simulink model "Autopilot_q_running1"  (R2021a)
settings: Solver=ode4  StartTime=0.0  StopTime=168  FixedStep=0.01  RelTol=1e-3
undefined symbols (not defined in the file or in its folder): Aero_cofficients, Earth, Plane_state_store, Structural_data, Thrust_data_store, WGS84
libraries: pid_lib x12, aerolibactuator x5, aerolibfltsims x2, aerolibanim x1, simulink x1, aerolibtransform2 x1, shared6dof x1, sim3dlib x1, uavsim3dlib x1
(part 1 of 3)
settings Model: PauseTimes=.01  Creator=rrpat  LastModifiedBy=PC
settings SolverCC: AlgebraicLoopSolver=LineSearch
settings DataIOCC: ReturnWorkspaceOutputs=off
settings DebuggingCC: SFMachineParentedDataDiag=warning  ArithmeticOperatorsInVariantConditions=warning
settings SFSimCC: CustomCodeUndefinedFunction=UseInterfaceOnly

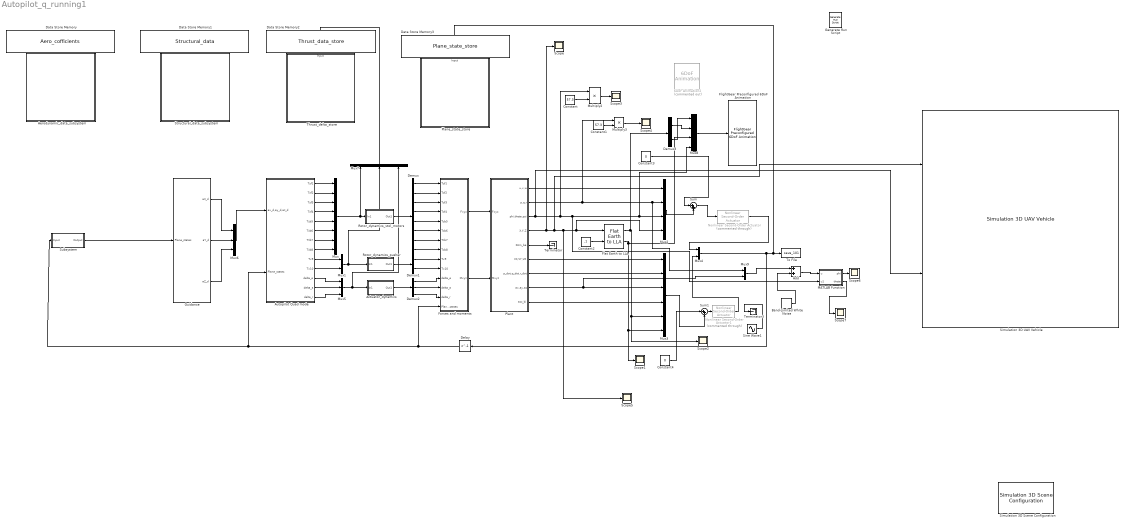
== system Autopilot_q_running1 ==
  6DoF Animation2 : aerolibanim/6DoF Animation  Commented=on  u1=[-150 150 -150 150 -150 150]  u2=0.1  u3=100  u4=[-4000 0 2000]  u5=Fly alongside  u6="[300  300 -200]"  u7=10  u8=on
  Actuator_dynamics : Subsystem
  Add : Sum
  Aerodynamic_data_subsystem : Subsystem
  Autopilot Quad mode : Subsystem
  Band-Limited White Noise : simulink/Sources/Band-Limited White Noise  Cov=[0.0001]  Ts=0.1  seed=[23341]
  Constant : Constant  Value=57.3
  Constant1 : Constant  Value=57.3
  Constant2 : Constant  Value=-7
  Constant3 : Constant  Value=0
  Constant4 : Constant  Value=0
  Data Store Memory : DataStoreMemory  DataStoreName=Aero_cofficients  ReadBeforeWriteMsg=warning  WriteAfterWriteMsg=warning  WriteAfterReadMsg=warning  InitialValue=[0 0 0 0 0 0 0 0 0;0 0 0 0 0 0 0 0 0;0 0 0 0 0 0 0 0 0;0 0 0 0 0 0 0 0 0;0 0 0 0 0 0 0 0 0;0 0 0 0 0 0 0 0 0]  ShareAcrossModelInstances=on  VectorParams1D=off  ShowAdditionalParam=off
  Data Store Memory1 : DataStoreMemory  DataStoreName=Structural_data  ReadBeforeWriteMsg=warning  WriteAfterWriteMsg=warning  WriteAfterReadMsg=warning  InitialValue=[25.0,0,0,0,0,0,0,0,0,0,0,0,0,0,0,0,0,0,0,0,0,0,0,0]  ShareAcrossModelInstances=on  VectorParams1D=off  ShowAdditionalParam=off
  Data Store Memory2 : DataStoreMemory  DataStoreName=Thrust_data_store  ReadBeforeWriteMsg=warning  WriteAfterWriteMsg=warning  WriteAfterReadMsg=warning  InitialValue=[0,0,0,0,0,0,0,0,0,0,0,0,0]  ShareAcrossModelInstances=on  VectorParams1D=off  ShowAdditionalParam=off
  Data Store Memory3 : DataStoreMemory  DataStoreName=Plane_state_store  ReadBeforeWriteMsg=warning  WriteAfterWriteMsg=warning  WriteAfterReadMsg=warning  InitialValue=[0.0,0,0,0,0,0,0,0,30/57.3,0,0,0,0,0,0,0,0,0,0,0,0,0,0,0,0,0,0]  ShareAcrossModelInstances=on  VectorParams1D=off  ShowAdditionalParam=off
  Delay : Delay  DelayLength=1
  Demux : Demux  Outputs=8
  Demux1 : Demux  Outputs=2
  Demux2 : Demux  Outputs=3
  Demux3 : Demux  Outputs=2
  Flat Earth to LLA : aerolibtransform2/Flat Earth to LLA  units=Metric (MKS)  ptype=Earth (WGS84)  F=1/298.257223563  R=6378137  refPosPort=off  LL0=[37.6188056,-122.3754167 ]  psi=0
  FlightGear Preconfigured 6DoF Animation : aerolibfltsims/FlightGear Preconfigured 6DoF Animation  xFlightGearVersion=v2016.3  DestinationIpAddress=127.0.0.1  DestinationPort=5502  SampleTime=0.01  packetVersion=24
  Forces and moments : Subsystem
  Generate Run Script : aerolibfltsims/Generate Run Script  Architecture=Default  dataFlow=Send  GeometryModelName=HL20  AirportId=KSFO  RunwayId=10L  InitialAltitude=500  InitialHeading=0  OffsetDistance=4.72  OffsetAzimuth=0  InstallScenery=on  DisableShaders=off  OriginAddress=127.0.0.1  DestinationPort=5502  OriginPort=5505  LocalAddress=127.0.0.1  OutputFileName=runfg.bat  FlightGearBaseDirectory=C:\Program Files\FlightGear 2016.3.1
  Guidance : Subsystem
  MATLAB Function : MATLAB Function  TreatAsAtomicUnit=on
  Multiply2 : Product
  Multiply3 : Product
  Mux : Mux  Inputs=8
  Mux1 : Mux  Inputs=2
  Mux2 : Mux
  Mux3 : Mux  Inputs=6
  Mux4 : Mux  Inputs=2
  Mux5 : Mux  Inputs=3
  Mux6 : Mux  Inputs=3
  Mux7 : Mux  Inputs=3
  Mux8 : Mux
  Mux9 : Mux  Inputs=2
  Nonlinear Second-Order Actuator : aerolibactuator/Nonlinear Second-Order Actuator  Commented=through  wn_fin=50  z_fin=0.5  fin_max=500000000  fin_min=-500000000  fin_maxrate=2  fin_act_0=0  fin_act_vel=0
      settings: SourceProductBaseCode=AE
  Nonlinear Second-Order Actuator1 : aerolibactuator/Nonlinear Second-Order Actuator  Commented=through  wn_fin=50  z_fin=0.5  fin_max=5000000  fin_min=-5000000  fin_maxrate=2  fin_act_0=0  fin_act_vel=0
      settings: SourceProductBaseCode=AE
  Plane_state_store : Subsystem
  Plant : Subsystem
  Rotor_dynamics_pusher : Subsystem
  Rotor_dynamics_vtol_motors : Subsystem
  Scope{,1..7} (8 alike) : Scope
  Simulation 3D Scene Configuration : sim3dlib/Simulation 3D Scene Configuration  Priority=0  ProjectFormat=Default Scenes  SceneDesc=US city block  ProjectName=C:\Program Files\MATLAB\R2021a\toolbox\shared\sim3d_projects\automotive_project\UE4\WindowsNoEditor\VehicleSimulation.exe  ScenePath=/Game/Maps/HwStrght  vehTagList={'Scene Origin';'SimulinkVehicle1'}  vehTag=SimulinkVehicle1  OpVisEn=off  Ts=0.01  EnableWindow=on  EnableWeather=off  SunAltitude=40.0  SunAzimuth=90  clouds=10  wind=1  fog=0  rain=0  sensorTag=MainCamera1  sensorId=1  sensorName=MainCamera1  mountLoc=Origin  offsetFlag=off  tmountOffset=[0, 0, 0]  rmountOffset=[0, 0, 0]  HorizontalResolution=1280  VerticalResolution=720  HorizontalFOV=60  mountPoint=[0 0 0]  mountOrientation=[0 0 0]  aMode=3  ID=1
      settings: SourceProductBaseCode=DR,UV,VE
  Simulation 3D UAV Vehicle : uavsim3dlib/Simulation 3D UAV Vehicle  Priority=-1  Mesh=Quadrotor  Color=Blue  ActorName=SimulinkVehicle1  InitialTranslation=[0 0 0]  InitialRotation=[0 0 0]  SampleTime=-1  ActorType=SimulinkVehicle  ID=1  aMode=4  ActorTag=SimulinkVehicle1
      settings: SourceProductBaseCode=UV
  Sine Wave1 : Sin  Amplitude=0.1/57.3  Frequency=100*2*3.1415  SampleTime=0
  Structural_data_subsystem : Subsystem
  Subsystem : Subsystem
  Sum : Sum  Inputs=|++
  Sum1 : Sum  Inputs=|++
  Terminator : Terminator
  Terminator3 : Terminator
  Thrust_delta_store : Subsystem
  To File : ToFile  Filename=save_101  SaveFormat=Timeseries
  wires:
  Constant2/1 -> Flat Earth to LLA/2
  Plant/4(X,Y,Z) -> Scope/1, Simulation 3D UAV Vehicle/1, Scope5/1, Mux2/4, Flat Earth to LLA/1
  Plant/5(Dcm_be) -> Terminator/1
  Plant/1(u,v,w) -> Mux2/1
  Plant/2(p,q,r) -> Multiply3/1, Mux9/1, Mux2/2
  Plant/3(phi,theta,psi) -> Simulation 3D UAV Vehicle/2, MATLAB Function/2(u1), Mux8/4, Mux2/3, Multiply2/1
  Plant/9(acc_bi) -> Mux3/4
  Plant/8(ax,ay,az) -> Mux9/2, Mux3/3
  Plant/7(p_dot,q_dot,r_dot) -> Mux3/2
  Plant/6(VX,VY,VZ) -> Mux3/1
  Forces and moments/2(Mxyz) -> Plant/2(Mxyz)
  Flat Earth to LLA/1 -> Demux3/1, Mux3/5, Scope2/1
  Flat Earth to LLA/2 -> Mux8/3, Mux3/6, Scope1/1
  Autopilot Quad mode/1(Tzf1) -> Mux/1
  Autopilot Quad mode/2(Tzf2) -> Mux/2
  Autopilot Quad mode/3(Tzf3) -> Mux/3
  Autopilot Quad mode/4(Tzf4) -> Mux/4
  Autopilot Quad mode/5(Tzb5) -> Mux/5
  Autopilot Quad mode/6(Tzb6) -> Mux/6
  Autopilot Quad mode/7(Tzb7) -> Mux/7
  Autopilot Quad mode/8(Tzb8) -> Mux/8
  Demux/8 -> Forces and moments/8(Tzb8)
  Demux/7 -> Forces and moments/7(Tzb7)
  Demux/1 -> Forces and moments/1(Tzf1)
  Demux/3 -> Forces and moments/3("Tzf3 ")
  Demux/4 -> Forces and moments/4(Tzf4)
  Demux/5 -> Forces and moments/5(Tzb5)
  Demux/6 -> Forces and moments/6(Tzb6)
  Demux1/1 -> Forces and moments/9(Tx9)
  Demux1/2 -> Forces and moments/10(Tx10)
  Rotor_dynamics_pusher/1(Out1) -> Demux1/1
  Autopilot Quad mode/9(Tx9) -> Mux1/1
  Autopilot Quad mode/10(Tx10) -> Mux1/2
  Demux2/1 -> Forces and moments/11(delta_e)
  Demux2/2 -> Forces and moments/12(delta_a)
  Demux2/3 -> Forces and moments/13(delta_r)
  Actuator_dynamics/1(Out1) -> Demux2/1
  Autopilot Quad mode/11(delta_e) -> Mux5/1
  Autopilot Quad mode/12(delta_a) -> Mux5/2
  Autopilot Quad mode/13(delta_r) -> Mux5/3
  Rotor_dynamics_vtol_motors/1(Out1) -> Demux/1
  Forces and moments/1(Fxyz) -> Plant/1(Fxyz)
  Guidance/1(aX_d) -> Mux6/1
  Guidance/3(aZ_d) -> Mux6/3
  Guidance/2(aY_d) -> Mux6/2
  Mux6/1 -> Autopilot Quad mode/1(ax_d,ay_d,az_d)
  Mux/1 -> Mux7/1, Rotor_dynamics_vtol_motors/1(In1)
  Mux1/1 -> Rotor_dynamics_pusher/1(In1), Mux7/2
  Mux5/1 -> Actuator_dynamics/1(In1), Mux7/3
  Subsystem/1(Output) -> Guidance/1(Plane_states)
  Mux7/1 -> Thrust_delta_store/1(Input)
  Constant/1 -> Multiply2/2
  Multiply2/1 -> Scope3/1
  Constant1/1 -> Multiply3/2
  Multiply3/1 -> Scope4/1
  Mux3/1 -> Sum1/2
  Mux2/1 -> Sum/2
  Sine Wave1/1 -> Terminator3/1
  Sum/1 -> Nonlinear Second-Order Actuator/1
  Mux4/1 -> Plane_state_store/1(Input), To File/1, Delay/1
  Sum1/1 -> Nonlinear Second-Order Actuator1/1
  Nonlinear Second-Order Actuator/1 -> Mux4/1
  Nonlinear Second-Order Actuator1/1 -> Mux4/2
  Mux8/1 -> FlightGear Preconfigured 6DoF Animation/1
  Demux3/1 -> Mux8/2
  Constant3/1 -> Sum/1
  Constant4/1 -> Sum1/1
  Demux/2 -> Forces and moments/2(Tzf2)
  Demux3/2 -> Mux8/1
  Mux9/1 -> Add/1
  Band-Limited White Noise/1 -> Add/2
  Add/1 -> MATLAB Function/1(u)
  MATLAB Function/1(phi) -> Scope6/1
  MATLAB Function/2(theta) -> Scope7/1
  Delay/1 -> Subsystem/1(Input), Autopilot Quad mode/2(Plane_states), Forces and moments/14(Plane_states)

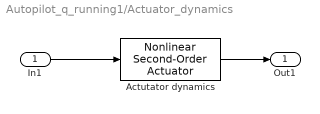
== system Autopilot_q_running1/Actuator_dynamics ==
  In1 : Inport
  Actutator dynamics : aerolibactuator/Nonlinear Second-Order Actuator  wn_fin=100  z_fin=0.3  fin_max=20*pi/180  fin_min=-20*pi/180  fin_maxrate=500*pi/180  fin_act_0=0  fin_act_vel=0
      settings: SourceProductBaseCode=AE
  Out1 : Outport  VectorParamsAs1DForOutWhenUnconnected=off
  wires:
  Actutator dynamics/1 -> Out1/1
  In1/1 -> Actutator dynamics/1

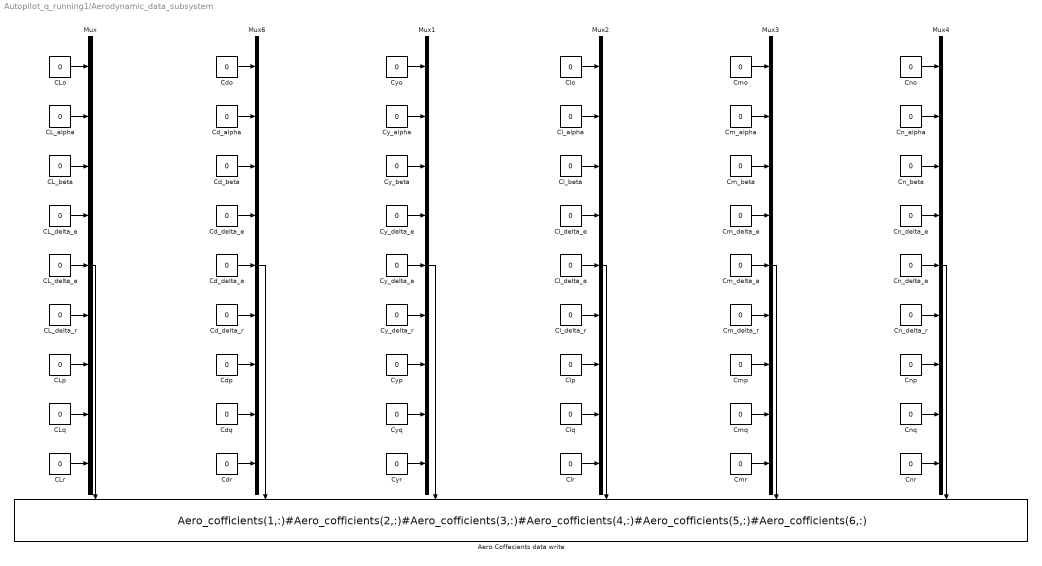
== system Autopilot_q_running1/Aerodynamic_data_subsystem ==
  Aero Coffecients data write : DataStoreWrite  DataStoreName=Aero_cofficients  DataStoreElements=Aero_cofficients(1,:)#Aero_cofficients(2,:)#Aero_cofficients(3,:)#Aero_cofficients(4,:)#Aero_cofficients(5,:)#Aero_cofficients(6,:)  IndexOptions=Index vector (dialog)  Indices=1  OutputSizes=1
  CL_alpha : Constant  Value=0
  CL_beta : Constant  Value=0
  CL_delta_a : Constant  Value=0
  CL_delta_e : Constant  Value=0
  CL_delta_r : Constant  Value=0
  CLo : Constant  Value=0
  CLp : Constant  Value=0
  CLq : Constant  Value=0
  CLr : Constant  Value=0
  Cd_alpha : Constant  Value=0
  Cd_beta : Constant  Value=0
  Cd_delta_a : Constant  Value=0
  Cd_delta_e : Constant  Value=0
  Cd_delta_r : Constant  Value=0
  Cdo : Constant  Value=0
  Cdp : Constant  Value=0
  Cdq : Constant  Value=0
  Cdr : Constant  Value=0
  Cl_alpha : Constant  Value=0
  Cl_beta : Constant  Value=0
  Cl_delta_a : Constant  Value=0
  Cl_delta_e : Constant  Value=0
  Cl_delta_r : Constant  Value=0
  Clo : Constant  Value=0
  Clp : Constant  Value=0
  Clq : Constant  Value=0
  Clr : Constant  Value=0
  Cm_alpha : Constant  Value=0
  Cm_beta : Constant  Value=0
  Cm_delta_a : Constant  Value=0
  Cm_delta_e : Constant  Value=0
  Cm_delta_r : Constant  Value=0
  Cmo : Constant  Value=0
  Cmp : Constant  Value=0
  Cmq : Constant  Value=0
  Cmr : Constant  Value=0
  Cn_alpha : Constant  Value=0
  Cn_beta : Constant  Value=0
  Cn_delta_a : Constant  Value=0
  Cn_delta_e : Constant  Value=0
  Cn_delta_r : Constant  Value=0
  Cno : Constant  Value=0
  Cnp : Constant  Value=0
  Cnq : Constant  Value=0
  Cnr : Constant  Value=0
  Cy_alpha : Constant  Value=0
  Cy_beta : Constant  Value=0
  Cy_delta_a : Constant  Value=0
  Cy_delta_e : Constant  Value=0
  Cy_delta_r : Constant  Value=0
  Cyo : Constant  Value=0
  Cyp : Constant  Value=0
  Cyq : Constant  Value=0
  Cyr : Constant  Value=0
  Mux{,1..4,6} (6 alike) : Mux  Inputs=9
  wires:
  Mux/1 -> Aero Coffecients data write/1
  CLo/1 -> Mux/1
  CL_alpha/1 -> Mux/2
  CL_beta/1 -> Mux/3
  CL_delta_e/1 -> Mux/4
  CL_delta_a/1 -> Mux/5
  CL_delta_r/1 -> Mux/6
  CLp/1 -> Mux/7
  CLq/1 -> Mux/8
  CLr/1 -> Mux/9
  Cdo/1 -> Mux6/1
  Cd_delta_e/1 -> Mux6/4
  Cdq/1 -> Mux6/8
  Cdp/1 -> Mux6/7
  Cd_delta_a/1 -> Mux6/5
  Cdr/1 -> Mux6/9
  Cd_beta/1 -> Mux6/3
  Cd_delta_r/1 -> Mux6/6
  Cd_alpha/1 -> Mux6/2
  Mux6/1 -> Aero Coffecients data write/2
  Cy_alpha/1 -> Mux1/2
  Cy_delta_r/1 -> Mux1/6
  Cy_beta/1 -> Mux1/3
  Cyr/1 -> Mux1/9
  Cy_delta_a/1 -> Mux1/5
  Cyp/1 -> Mux1/7
  Cyq/1 -> Mux1/8
  Cy_delta_e/1 -> Mux1/4
  Cyo/1 -> Mux1/1
  Mux1/1 -> Aero Coffecients data write/3
  Mux2/1 -> Aero Coffecients data write/4
  Clo/1 -> Mux2/1
  Cl_delta_e/1 -> Mux2/4
  Clq/1 -> Mux2/8
  Clp/1 -> Mux2/7
  Cl_delta_a/1 -> Mux2/5
  Clr/1 -> Mux2/9
  Cl_beta/1 -> Mux2/3
  Cl_delta_r/1 -> Mux2/6
  Cl_alpha/1 -> Mux2/2
  Mux3/1 -> Aero Coffecients data write/5
  Cmo/1 -> Mux3/1
  Cm_delta_e/1 -> Mux3/4
  Cmq/1 -> Mux3/8
  Cmp/1 -> Mux3/7
  Cm_delta_a/1 -> Mux3/5
  Cmr/1 -> Mux3/9
  Cm_beta/1 -> Mux3/3
  Cm_delta_r/1 -> Mux3/6
  Cm_alpha/1 -> Mux3/2
  Mux4/1 -> Aero Coffecients data write/6
  Cno/1 -> Mux4/1
  Cn_delta_e/1 -> Mux4/4
  Cnq/1 -> Mux4/8
  Cnp/1 -> Mux4/7
  Cn_delta_a/1 -> Mux4/5
  Cnr/1 -> Mux4/9
  Cn_beta/1 -> Mux4/3
  Cn_delta_r/1 -> Mux4/6
  Cn_alpha/1 -> Mux4/2

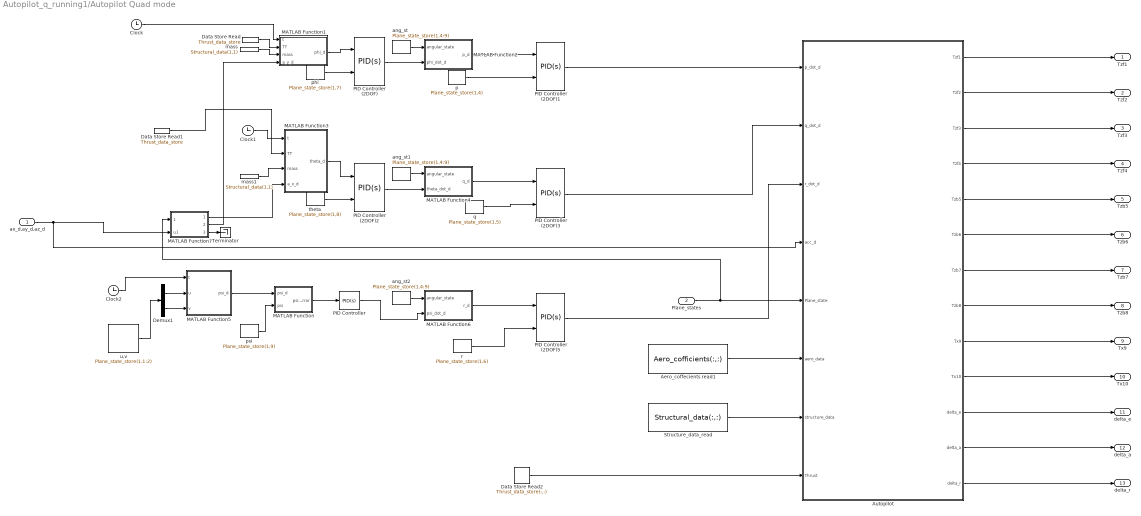
== system Autopilot_q_running1/Autopilot Quad mode ==
  ax_d,ay_d,az_d : Inport
  Plane_states : Inport  Port=2
  Aero_coffecients read1 : DataStoreRead  DataStoreName=Aero_cofficients  DataStoreElements=Aero_cofficients(:,:)  IndexOptions=Index vector (dialog)  Indices=1  OutputSizes=1
  Autopilot : MATLAB Function  TreatAsAtomicUnit=on
  Clock : Clock
      settings: Decimation=200
  Clock1 : Clock
      settings: Decimation=200
  Clock2 : Clock
      settings: Decimation=200
  Data Store Read : DataStoreRead  DataStoreName=Thrust_data_store  IndexOptions=Index vector (dialog)  Indices=1  OutputSizes=1
  Data Store Read1 : DataStoreRead  DataStoreName=Thrust_data_store  IndexOptions=Index vector (dialog)  Indices=1  OutputSizes=1
  Data Store Read2 : DataStoreRead  DataStoreName=Thrust_data_store  DataStoreElements=Thrust_data_store(:,:)  IndexOptions=Index vector (dialog)  Indices=1  OutputSizes=1
  Demux1 : Demux  Outputs=2
  MATLAB Function : MATLAB Function  TreatAsAtomicUnit=on
  MATLAB Function1 : MATLAB Function  TreatAsAtomicUnit=on
  MATLAB Function2 : MATLAB Function  TreatAsAtomicUnit=on
  MATLAB Function3 : MATLAB Function  TreatAsAtomicUnit=on
  MATLAB Function4 : MATLAB Function  TreatAsAtomicUnit=on
  MATLAB Function5 : MATLAB Function  TreatAsAtomicUnit=on
  MATLAB Function6 : MATLAB Function  TreatAsAtomicUnit=on
  MATLAB Function7 : MATLAB Function  TreatAsAtomicUnit=on
  PID Controller : pid_lib/PID Controller  Controller=PID  Form=Parallel  TimeDomain=Continuous-time  UseExternalTs=off  SampleTime=-1  IntegratorMethod=Forward Euler  FilterMethod=Forward Euler  ControllerParametersSource=internal  P=1  I=0  D=0  UseFilter=on  N=100  TunerSelectOption=Transfer Function Based (PID Tuner App)  InitialConditionSource=internal  InitialConditionForIntegrator=0  InitialConditionForFilter=0  DifferentiatorICPrevScaledInput=0  ExternalReset=none  TrackingMode=off  Kt=1  LimitOutput=off  SatLimitsSource=internal  UpperSaturationLimit=inf  LowerSaturationLimit=-inf  LinearizeAsGain=on  AntiWindupMode=none  Kb=1  POutMin=[]  POutMax=[]  IOutMin=[]  IOutMax=[]  DOutMin=[]  DOutMax=[]  NOutMin=[]  NOutMax=[]  SumOutMin=[]  SumOutMax=[]  SaturationOutMin=[]  SaturationOutMax=[]  PParamMin=[]  PParamMax=[]  IParamMin=[]  IParamMax=[]  DParamMin=[]  DParamMax=[]  NParamMin=[]  NParamMax=[]  KbParamMin=[]  KbParamMax=[]  KtParamMin=[]  KtParamMax=[]  KbOutMin=[]  KbOutMax=[]  KtOutMin=[]  KtOutMax=[]  IntegratorOutMin=[]  IntegratorOutMax=[]  FilterOutMin=[]  FilterOutMax=[]  SumI1OutMin=[]  SumI1OutMax=[]  SumI2OutMin=[]  SumI2OutMax=[]  SumI3OutMin=[]  SumI3OutMax=[]  SumI4OutMin=[]  SumI4OutMax=[]  SumDOutMin=[]  SumDOutMax=[]  DifferentiatorOutMin=[]  DifferentiatorOutMax=[]  FilterDiffOutCoefMin=[]  FilterDiffOutCoefMax=[]  ReciprocalOutMin=[]  ReciprocalOutMax=[]  SumDenOutMin=[]  SumDenOutMax=[]  SumNumOutMin=[]  SumNumOutMax=[]  DivideOutMin=[]  DivideOutMax=[]  UdiffTsProdOutMin=[]  UdiffTsProdOutMax=[]  NTsProdOutMin=[]  NTsProdOutMax=[]  UintegralTsProdOutMin=[]  UintegralTsProdOutMax=[]  UngainTsProdOutMin=[]  UngainTsProdOutMax=[]  IntegratorContinuousStateAttributes=''  IntegratorStateMustResolveToSignalObject=off  IntegratorRTWStateStorageClass=Auto  FilterContinuousStateAttributes=''  FilterStateMustResolveToSignalObject=off  FilterRTWStateStorageClass=Auto  ParallelPVariant=InternalParameters  IdealPVariant=Disabled  IVariant=InternalParameters  DVariant=InternalParameters  IntegratorVariant=Continuous  SatVariant=Disabled  AWVariant=Passthrough  PCopyVariant=Disabled  TRVariant=Disabled  FdbkBlocksVariant=Forward  IdealPFdbkVariant=Disabled  SatFdbkVariant=Disabled  DerivativeFilterVariant=ContFilter  NVariant=InternalParameters  NCopyVariant=Disabled  FilterICVariant=InternalICsFilter  IntegratorICVariant=InternalICs  ExternalResetVariant=Disabled  TRSumVariant=Passthrough  SumFdbkVariant=Disabled  SumVariant=Sum_PID  TsampFilterVariant=InternalTs  TsampNgainVariant=Passthrough  TsampIntegralVariant=Passthrough  ExternalSaturationOutDataTypeStr=Inherit: Same as second input
  PID Controller (2DOF) : pid_lib/PID Controller (2DOF)  Controller=PID  Form=Parallel  TimeDomain=Continuous-time  UseExternalTs=off  SampleTime=-1  IntegratorMethod=Forward Euler  FilterMethod=Forward Euler  ControllerParametersSource=internal  P=1  I=0  D=0  UseFilter=on  N=100  b=1  c=1  TunerSelectOption=Transfer Function Based (PID Tuner App)  InitialConditionSource=internal  InitialConditionForIntegrator=0  InitialConditionForFilter=0  DifferentiatorICPrevScaledInput=0  ExternalReset=none  TrackingMode=off  Kt=1  LimitOutput=off  SatLimitsSource=internal  UpperSaturationLimit=inf  LowerSaturationLimit=-inf  LinearizeAsGain=on  AntiWindupMode=none  Kb=1  POutMin=[]  POutMax=[]  IOutMin=[]  IOutMax=[]  DOutMin=[]  DOutMax=[]  NOutMin=[]  NOutMax=[]  bOutMin=[]  bOutMax=[]  cOutMin=[]  cOutMax=[]  SumOutMin=[]  SumOutMax=[]  SaturationOutMin=[]  SaturationOutMax=[]  PParamMin=[]  PParamMax=[]  IParamMin=[]  IParamMax=[]  DParamMin=[]  DParamMax=[]  NParamMin=[]  NParamMax=[]  bParamMin=[]  bParamMax=[]  cParamMin=[]  cParamMax=[]  KbParamMin=[]  KbParamMax=[]  KtParamMin=[]  KtParamMax=[]  KbOutMin=[]  KbOutMax=[]  KtOutMin=[]  KtOutMax=[]  IntegratorOutMin=[]  IntegratorOutMax=[]  FilterOutMin=[]  FilterOutMax=[]  SumI1OutMin=[]  SumI1OutMax=[]  SumI2OutMin=[]  SumI2OutMax=[]  SumI3OutMin=[]  SumI3OutMax=[]  SumI4OutMin=[]  SumI4OutMax=[]  SumDOutMin=[]  SumDOutMax=[]  Sum1OutMin=[]  Sum1OutMax=[]  Sum2OutMin=[]  Sum2OutMax=[]  Sum3OutMin=[]  Sum3OutMax=[]  DifferentiatorOutMin=[]  DifferentiatorOutMax=[]  FilterDiffOutCoefMin=[]  FilterDiffOutCoefMax=[]  ReciprocalOutMin=[]  ReciprocalOutMax=[]  SumDenOutMin=[]  SumDenOutMax=[]  SumNumOutMin=[]  SumNumOutMax=[]  DivideOutMin=[]  DivideOutMax=[]  UdiffTsProdOutMin=[]  UdiffTsProdOutMax=[]  NTsProdOutMin=[]  NTsProdOutMax=[]  UintegralTsProdOutMin=[]  UintegralTsProdOutMax=[]  UngainTsProdOutMin=[]  UngainTsProdOutMax=[]  IntegratorContinuousStateAttributes=''  IntegratorStateMustResolveToSignalObject=off  IntegratorRTWStateStorageClass=Auto  FilterContinuousStateAttributes=''  FilterStateMustResolveToSignalObject=off  FilterRTWStateStorageClass=Auto  ParallelPVariant=InternalParameters  IdealPVariant=Disabled  IVariant=InternalParameters  DVariant=InternalParameters  bVariant=InternalParameters  cVariant=InternalParameters  IntegratorVariant=Continuous  SatVariant=Disabled  AWVariant=Passthrough  PCopyVariant=Disabled  TRVariant=Disabled  FdbkBlocksVariant=Forward  IdealPFdbkVariant=Disabled  SatFdbkVariant=Disabled  DerivativeFilterVariant=ContFilter  NVariant=InternalParameters  NCopyVariant=Disabled  FilterICVariant=InternalICsFilter  IntegratorICVariant=InternalICs  ExternalResetVariant=Disabled  TRSumVariant=Passthrough  SumFdbkVariant=Disabled  SumVariant=Sum_PID  TsampFilterVariant=InternalTs  TsampNgainVariant=Passthrough  TsampIntegralVariant=Passthrough  ExternalSaturationOutDataTypeStr=Inherit: Same as second input
      settings: SourceProductBaseCode=SL
  PID Controller (2DOF)1 : pid_lib/PID Controller (2DOF)  Controller=PID  Form=Parallel  TimeDomain=Continuous-time  UseExternalTs=off  SampleTime=-1  IntegratorMethod=Forward Euler  FilterMethod=Forward Euler  ControllerParametersSource=internal  P=3  I=0.1  D=0  UseFilter=on  N=100  b=1  c=1  TunerSelectOption=Transfer Function Based (PID Tuner App)  InitialConditionSource=internal  InitialConditionForIntegrator=0  InitialConditionForFilter=0  DifferentiatorICPrevScaledInput=0  ExternalReset=none  TrackingMode=off  Kt=1  LimitOutput=off  SatLimitsSource=internal  UpperSaturationLimit=inf  LowerSaturationLimit=-inf  LinearizeAsGain=on  AntiWindupMode=none  Kb=1  POutMin=[]  POutMax=[]  IOutMin=[]  IOutMax=[]  DOutMin=[]  DOutMax=[]  NOutMin=[]  NOutMax=[]  bOutMin=[]  bOutMax=[]  cOutMin=[]  cOutMax=[]  SumOutMin=[]  SumOutMax=[]  SaturationOutMin=[]  SaturationOutMax=[]  PParamMin=[]  PParamMax=[]  IParamMin=[]  IParamMax=[]  DParamMin=[]  DParamMax=[]  NParamMin=[]  NParamMax=[]  bParamMin=[]  bParamMax=[]  cParamMin=[]  cParamMax=[]  KbParamMin=[]  KbParamMax=[]  KtParamMin=[]  KtParamMax=[]  KbOutMin=[]  KbOutMax=[]  KtOutMin=[]  KtOutMax=[]  IntegratorOutMin=[]  IntegratorOutMax=[]  FilterOutMin=[]  FilterOutMax=[]  SumI1OutMin=[]  SumI1OutMax=[]  SumI2OutMin=[]  SumI2OutMax=[]  SumI3OutMin=[]  SumI3OutMax=[]  SumI4OutMin=[]  SumI4OutMax=[]  SumDOutMin=[]  SumDOutMax=[]  Sum1OutMin=[]  Sum1OutMax=[]  Sum2OutMin=[]  Sum2OutMax=[]  Sum3OutMin=[]  Sum3OutMax=[]  DifferentiatorOutMin=[]  DifferentiatorOutMax=[]  FilterDiffOutCoefMin=[]  FilterDiffOutCoefMax=[]  ReciprocalOutMin=[]  ReciprocalOutMax=[]  SumDenOutMin=[]  SumDenOutMax=[]  SumNumOutMin=[]  SumNumOutMax=[]  DivideOutMin=[]  DivideOutMax=[]  UdiffTsProdOutMin=[]  UdiffTsProdOutMax=[]  NTsProdOutMin=[]  NTsProdOutMax=[]  UintegralTsProdOutMin=[]  UintegralTsProdOutMax=[]  UngainTsProdOutMin=[]  UngainTsProdOutMax=[]  IntegratorContinuousStateAttributes=''  IntegratorStateMustResolveToSignalObject=off  IntegratorRTWStateStorageClass=Auto  FilterContinuousStateAttributes=''  FilterStateMustResolveToSignalObject=off  FilterRTWStateStorageClass=Auto  ParallelPVariant=InternalParameters  IdealPVariant=Disabled  IVariant=InternalParameters  DVariant=InternalParameters  bVariant=InternalParameters  cVariant=InternalParameters  IntegratorVariant=Continuous  SatVariant=Disabled  AWVariant=Passthrough  PCopyVariant=Disabled  TRVariant=Disabled  FdbkBlocksVariant=Forward  IdealPFdbkVariant=Disabled  SatFdbkVariant=Disabled  DerivativeFilterVariant=ContFilter  NVariant=InternalParameters  NCopyVariant=Disabled  FilterICVariant=InternalICsFilter  IntegratorICVariant=InternalICs  ExternalResetVariant=Disabled  TRSumVariant=Passthrough  SumFdbkVariant=Disabled  SumVariant=Sum_PID  TsampFilterVariant=InternalTs  TsampNgainVariant=Passthrough  TsampIntegralVariant=Passthrough  ExternalSaturationOutDataTypeStr=Inherit: Same as second input
      settings: SourceProductBaseCode=SL
  PID Controller (2DOF)2 : pid_lib/PID Controller (2DOF)  Controller=PID  Form=Parallel  TimeDomain=Continuous-time  UseExternalTs=off  SampleTime=-1  IntegratorMethod=Forward Euler  FilterMethod=Forward Euler  ControllerParametersSource=internal  P=1  I=0  D=0  UseFilter=on  N=100  b=1  c=1  TunerSelectOption=Transfer Function Based (PID Tuner App)  InitialConditionSource=internal  InitialConditionForIntegrator=0  InitialConditionForFilter=0  DifferentiatorICPrevScaledInput=0  ExternalReset=none  TrackingMode=off  Kt=1  LimitOutput=off  SatLimitsSource=internal  UpperSaturationLimit=inf  LowerSaturationLimit=-inf  LinearizeAsGain=on  AntiWindupMode=none  Kb=1  POutMin=[]  POutMax=[]  IOutMin=[]  IOutMax=[]  DOutMin=[]  DOutMax=[]  NOutMin=[]  NOutMax=[]  bOutMin=[]  bOutMax=[]  cOutMin=[]  cOutMax=[]  SumOutMin=[]  SumOutMax=[]  SaturationOutMin=[]  SaturationOutMax=[]  PParamMin=[]  PParamMax=[]  IParamMin=[]  IParamMax=[]  DParamMin=[]  DParamMax=[]  NParamMin=[]  NParamMax=[]  bParamMin=[]  bParamMax=[]  cParamMin=[]  cParamMax=[]  KbParamMin=[]  KbParamMax=[]  KtParamMin=[]  KtParamMax=[]  KbOutMin=[]  KbOutMax=[]  KtOutMin=[]  KtOutMax=[]  IntegratorOutMin=[]  IntegratorOutMax=[]  FilterOutMin=[]  FilterOutMax=[]  SumI1OutMin=[]  SumI1OutMax=[]  SumI2OutMin=[]  SumI2OutMax=[]  SumI3OutMin=[]  SumI3OutMax=[]  SumI4OutMin=[]  SumI4OutMax=[]  SumDOutMin=[]  SumDOutMax=[]  Sum1OutMin=[]  Sum1OutMax=[]  Sum2OutMin=[]  Sum2OutMax=[]  Sum3OutMin=[]  Sum3OutMax=[]  DifferentiatorOutMin=[]  DifferentiatorOutMax=[]  FilterDiffOutCoefMin=[]  FilterDiffOutCoefMax=[]  ReciprocalOutMin=[]  ReciprocalOutMax=[]  SumDenOutMin=[]  SumDenOutMax=[]  SumNumOutMin=[]  SumNumOutMax=[]  DivideOutMin=[]  DivideOutMax=[]  UdiffTsProdOutMin=[]  UdiffTsProdOutMax=[]  NTsProdOutMin=[]  NTsProdOutMax=[]  UintegralTsProdOutMin=[]  UintegralTsProdOutMax=[]  UngainTsProdOutMin=[]  UngainTsProdOutMax=[]  IntegratorContinuousStateAttributes=''  IntegratorStateMustResolveToSignalObject=off  IntegratorRTWStateStorageClass=Auto  FilterContinuousStateAttributes=''  FilterStateMustResolveToSignalObject=off  FilterRTWStateStorageClass=Auto  ParallelPVariant=InternalParameters  IdealPVariant=Disabled  IVariant=InternalParameters  DVariant=InternalParameters  bVariant=InternalParameters  cVariant=InternalParameters  IntegratorVariant=Continuous  SatVariant=Disabled  AWVariant=Passthrough  PCopyVariant=Disabled  TRVariant=Disabled  FdbkBlocksVariant=Forward  IdealPFdbkVariant=Disabled  SatFdbkVariant=Disabled  DerivativeFilterVariant=ContFilter  NVariant=InternalParameters  NCopyVariant=Disabled  FilterICVariant=InternalICsFilter  IntegratorICVariant=InternalICs  ExternalResetVariant=Disabled  TRSumVariant=Passthrough  SumFdbkVariant=Disabled  SumVariant=Sum_PID  TsampFilterVariant=InternalTs  TsampNgainVariant=Passthrough  TsampIntegralVariant=Passthrough  ExternalSaturationOutDataTypeStr=Inherit: Same as second input
      settings: SourceProductBaseCode=SL
  PID Controller (2DOF)3 : pid_lib/PID Controller (2DOF)  Controller=PID  Form=Parallel  TimeDomain=Continuous-time  UseExternalTs=off  SampleTime=-1  IntegratorMethod=Forward Euler  FilterMethod=Forward Euler  ControllerParametersSource=internal  P=3  I=0.1  D=0  UseFilter=on  N=100  b=1  c=1  TunerSelectOption=Transfer Function Based (PID Tuner App)  InitialConditionSource=internal  InitialConditionForIntegrator=0  InitialConditionForFilter=0  DifferentiatorICPrevScaledInput=0  ExternalReset=none  TrackingMode=off  Kt=1  LimitOutput=off  SatLimitsSource=internal  UpperSaturationLimit=inf  LowerSaturationLimit=-inf  LinearizeAsGain=on  AntiWindupMode=none  Kb=1  POutMin=[]  POutMax=[]  IOutMin=[]  IOutMax=[]  DOutMin=[]  DOutMax=[]  NOutMin=[]  NOutMax=[]  bOutMin=[]  bOutMax=[]  cOutMin=[]  cOutMax=[]  SumOutMin=[]  SumOutMax=[]  SaturationOutMin=[]  SaturationOutMax=[]  PParamMin=[]  PParamMax=[]  IParamMin=[]  IParamMax=[]  DParamMin=[]  DParamMax=[]  NParamMin=[]  NParamMax=[]  bParamMin=[]  bParamMax=[]  cParamMin=[]  cParamMax=[]  KbParamMin=[]  KbParamMax=[]  KtParamMin=[]  KtParamMax=[]  KbOutMin=[]  KbOutMax=[]  KtOutMin=[]  KtOutMax=[]  IntegratorOutMin=[]  IntegratorOutMax=[]  FilterOutMin=[]  FilterOutMax=[]  SumI1OutMin=[]  SumI1OutMax=[]  SumI2OutMin=[]  SumI2OutMax=[]  SumI3OutMin=[]  SumI3OutMax=[]  SumI4OutMin=[]  SumI4OutMax=[]  SumDOutMin=[]  SumDOutMax=[]  Sum1OutMin=[]  Sum1OutMax=[]  Sum2OutMin=[]  Sum2OutMax=[]  Sum3OutMin=[]  Sum3OutMax=[]  DifferentiatorOutMin=[]  DifferentiatorOutMax=[]  FilterDiffOutCoefMin=[]  FilterDiffOutCoefMax=[]  ReciprocalOutMin=[]  ReciprocalOutMax=[]  SumDenOutMin=[]  SumDenOutMax=[]  SumNumOutMin=[]  SumNumOutMax=[]  DivideOutMin=[]  DivideOutMax=[]  UdiffTsProdOutMin=[]  UdiffTsProdOutMax=[]  NTsProdOutMin=[]  NTsProdOutMax=[]  UintegralTsProdOutMin=[]  UintegralTsProdOutMax=[]  UngainTsProdOutMin=[]  UngainTsProdOutMax=[]  IntegratorContinuousStateAttributes=''  IntegratorStateMustResolveToSignalObject=off  IntegratorRTWStateStorageClass=Auto  FilterContinuousStateAttributes=''  FilterStateMustResolveToSignalObject=off  FilterRTWStateStorageClass=Auto  ParallelPVariant=InternalParameters  IdealPVariant=Disabled  IVariant=InternalParameters  DVariant=InternalParameters  bVariant=InternalParameters  cVariant=InternalParameters  IntegratorVariant=Continuous  SatVariant=Disabled  AWVariant=Passthrough  PCopyVariant=Disabled  TRVariant=Disabled  FdbkBlocksVariant=Forward  IdealPFdbkVariant=Disabled  SatFdbkVariant=Disabled  DerivativeFilterVariant=ContFilter  NVariant=InternalParameters  NCopyVariant=Disabled  FilterICVariant=InternalICsFilter  IntegratorICVariant=InternalICs  ExternalResetVariant=Disabled  TRSumVariant=Passthrough  SumFdbkVariant=Disabled  SumVariant=Sum_PID  TsampFilterVariant=InternalTs  TsampNgainVariant=Passthrough  TsampIntegralVariant=Passthrough  ExternalSaturationOutDataTypeStr=Inherit: Same as second input
      settings: SourceProductBaseCode=SL
  PID Controller (2DOF)5 : pid_lib/PID Controller (2DOF)  Controller=PID  Form=Parallel  TimeDomain=Continuous-time  UseExternalTs=off  SampleTime=-1  IntegratorMethod=Forward Euler  FilterMethod=Forward Euler  ControllerParametersSource=internal  P=3  I=0.1  D=0  UseFilter=on  N=100  b=1  c=1  TunerSelectOption=Transfer Function Based (PID Tuner App)  InitialConditionSource=internal  InitialConditionForIntegrator=0  InitialConditionForFilter=0  DifferentiatorICPrevScaledInput=0  ExternalReset=none  TrackingMode=off  Kt=1  LimitOutput=off  SatLimitsSource=internal  UpperSaturationLimit=inf  LowerSaturationLimit=-inf  LinearizeAsGain=on  AntiWindupMode=none  Kb=1  POutMin=[]  POutMax=[]  IOutMin=[]  IOutMax=[]  DOutMin=[]  DOutMax=[]  NOutMin=[]  NOutMax=[]  bOutMin=[]  bOutMax=[]  cOutMin=[]  cOutMax=[]  SumOutMin=[]  SumOutMax=[]  SaturationOutMin=[]  SaturationOutMax=[]  PParamMin=[]  PParamMax=[]  IParamMin=[]  IParamMax=[]  DParamMin=[]  DParamMax=[]  NParamMin=[]  NParamMax=[]  bParamMin=[]  bParamMax=[]  cParamMin=[]  cParamMax=[]  KbParamMin=[]  KbParamMax=[]  KtParamMin=[]  KtParamMax=[]  KbOutMin=[]  KbOutMax=[]  KtOutMin=[]  KtOutMax=[]  IntegratorOutMin=[]  IntegratorOutMax=[]  FilterOutMin=[]  FilterOutMax=[]  SumI1OutMin=[]  SumI1OutMax=[]  SumI2OutMin=[]  SumI2OutMax=[]  SumI3OutMin=[]  SumI3OutMax=[]  SumI4OutMin=[]  SumI4OutMax=[]  SumDOutMin=[]  SumDOutMax=[]  Sum1OutMin=[]  Sum1OutMax=[]  Sum2OutMin=[]  Sum2OutMax=[]  Sum3OutMin=[]  Sum3OutMax=[]  DifferentiatorOutMin=[]  DifferentiatorOutMax=[]  FilterDiffOutCoefMin=[]  FilterDiffOutCoefMax=[]  ReciprocalOutMin=[]  ReciprocalOutMax=[]  SumDenOutMin=[]  SumDenOutMax=[]  SumNumOutMin=[]  SumNumOutMax=[]  DivideOutMin=[]  DivideOutMax=[]  UdiffTsProdOutMin=[]  UdiffTsProdOutMax=[]  NTsProdOutMin=[]  NTsProdOutMax=[]  UintegralTsProdOutMin=[]  UintegralTsProdOutMax=[]  UngainTsProdOutMin=[]  UngainTsProdOutMax=[]  IntegratorContinuousStateAttributes=''  IntegratorStateMustResolveToSignalObject=off  IntegratorRTWStateStorageClass=Auto  FilterContinuousStateAttributes=''  FilterStateMustResolveToSignalObject=off  FilterRTWStateStorageClass=Auto  ParallelPVariant=InternalParameters  IdealPVariant=Disabled  IVariant=InternalParameters  DVariant=InternalParameters  bVariant=InternalParameters  cVariant=InternalParameters  IntegratorVariant=Continuous  SatVariant=Disabled  AWVariant=Passthrough  PCopyVariant=Disabled  TRVariant=Disabled  FdbkBlocksVariant=Forward  IdealPFdbkVariant=Disabled  SatFdbkVariant=Disabled  DerivativeFilterVariant=ContFilter  NVariant=InternalParameters  NCopyVariant=Disabled  FilterICVariant=InternalICsFilter  IntegratorICVariant=InternalICs  ExternalResetVariant=Disabled  TRSumVariant=Passthrough  SumFdbkVariant=Disabled  SumVariant=Sum_PID  TsampFilterVariant=InternalTs  TsampNgainVariant=Passthrough  TsampIntegralVariant=Passthrough  ExternalSaturationOutDataTypeStr=Inherit: Same as second input
      settings: SourceProductBaseCode=SL
  Structure_data_read : DataStoreRead  DataStoreName=Structural_data  DataStoreElements=Structural_data(:,:)  IndexOptions=Index vector (dialog)  Indices=1  OutputSizes=1
  Terminator : Terminator
  ang_st : DataStoreRead  DataStoreName=Plane_state_store  DataStoreElements=Plane_state_store(1,4:9)  IndexOptions=Index vector (dialog)  Indices=1  OutputSizes=1
  ang_st1 : DataStoreRead  DataStoreName=Plane_state_store  DataStoreElements=Plane_state_store(1,4:9)  IndexOptions=Index vector (dialog)  Indices=1  OutputSizes=1
  ang_st2 : DataStoreRead  DataStoreName=Plane_state_store  DataStoreElements=Plane_state_store(1,4:9)  IndexOptions=Index vector (dialog)  Indices=1  OutputSizes=1
  mass : DataStoreRead  DataStoreName=Structural_data  DataStoreElements=Structural_data(1,1)  IndexOptions=Index vector (dialog)  Indices=1  OutputSizes=1
  mass1 : DataStoreRead  DataStoreName=Structural_data  DataStoreElements=Structural_data(1,1)  IndexOptions=Index vector (dialog)  Indices=1  OutputSizes=1
  p : DataStoreRead  DataStoreName=Plane_state_store  DataStoreElements=Plane_state_store(1,4)  IndexOptions=Index vector (dialog)  Indices=1  OutputSizes=1
  phi : DataStoreRead  DataStoreName=Plane_state_store  DataStoreElements=Plane_state_store(1,7)  IndexOptions=Index vector (dialog)  Indices=1  OutputSizes=1
  psi : DataStoreRead  DataStoreName=Plane_state_store  DataStoreElements=Plane_state_store(1,9)  IndexOptions=Index vector (dialog)  Indices=1  OutputSizes=1
  "q " : DataStoreRead  DataStoreName=Plane_state_store  DataStoreElements=Plane_state_store(1,5)  IndexOptions=Index vector (dialog)  Indices=1  OutputSizes=1
  r : DataStoreRead  DataStoreName=Plane_state_store  DataStoreElements=Plane_state_store(1,6)  IndexOptions=Index vector (dialog)  Indices=1  OutputSizes=1
  theta : DataStoreRead  DataStoreName=Plane_state_store  DataStoreElements=Plane_state_store(1,8)  IndexOptions=Index vector (dialog)  Indices=1  OutputSizes=1
  u,v : DataStoreRead  DataStoreName=Plane_state_store  DataStoreElements=Plane_state_store(1,1:2)  IndexOptions=Index vector (dialog)  Indices=1  OutputSizes=1
  Tzf1 : Outport  VectorParamsAs1DForOutWhenUnconnected=off
  Tzf2 : Outport  Port=2  VectorParamsAs1DForOutWhenUnconnected=off
  Tzf3 : Outport  Port=3  VectorParamsAs1DForOutWhenUnconnected=off
  Tzf4 : Outport  Port=4  VectorParamsAs1DForOutWhenUnconnected=off
  Tzb5 : Outport  Port=5  VectorParamsAs1DForOutWhenUnconnected=off
  Tzb6 : Outport  Port=6  VectorParamsAs1DForOutWhenUnconnected=off
  Tzb7 : Outport  Port=7  VectorParamsAs1DForOutWhenUnconnected=off
  Tzb8 : Outport  Port=8  VectorParamsAs1DForOutWhenUnconnected=off
  Tx9 : Outport  Port=9  VectorParamsAs1DForOutWhenUnconnected=off
  Tx10 : Outport  Port=10  VectorParamsAs1DForOutWhenUnconnected=off
  delta_e : Outport  Port=11  VectorParamsAs1DForOutWhenUnconnected=off
  delta_a : Outport  Port=12  VectorParamsAs1DForOutWhenUnconnected=off
  delta_r : Outport  Port=13  VectorParamsAs1DForOutWhenUnconnected=off
  wires:
  Autopilot/4(Tzf4) -> Tzf4/1
  Autopilot/5(Tzb5) -> Tzb5/1
  Autopilot/6(Tzb6) -> Tzb6/1
  Autopilot/7(Tzb7) -> Tzb7/1
  Autopilot/8(Tzb8) -> Tzb8/1
  Autopilot/9(Tx9) -> Tx9/1
  Autopilot/10(Tx10) -> Tx10/1
  Autopilot/1(Tzf1) -> Tzf1/1
  Autopilot/2(Tzf2) -> Tzf2/1
  Autopilot/3(Tzf3) -> Tzf3/1
  Autopilot/11(delta_e) -> delta_e/1
  Autopilot/12(delta_a) -> delta_a/1
  Autopilot/13(delta_r) -> delta_r/1
  ax_d,ay_d,az_d/1 -> Autopilot/4(acc_d), MATLAB Function7/2(u1)
  Plane_states/1 -> MATLAB Function7/1(Plane_state), Autopilot/5(Plane_state)
  mass/1 -> MATLAB Function1/3(mass)
  MATLAB Function1/1(phi_d) -> PID Controller (2DOF)/1
  Data Store Read/1 -> MATLAB Function1/2(TT)
  phi/1 -> PID Controller (2DOF)/2
  p/1 -> PID Controller (2DOF)1/2
  ang_st/1 -> MATLAB Function2/1(angular_state)
  PID Controller (2DOF)/1 -> MATLAB Function2/2(phi_dot_d)
  MATLAB Function2/1(p_d) -> PID Controller (2DOF)1/1
  PID Controller (2DOF)1/1 -> Autopilot/1(p_dot_d)
  MATLAB Function4/1(q_d) -> PID Controller (2DOF)3/1
  theta/1 -> PID Controller (2DOF)2/2
  PID Controller (2DOF)2/1 -> MATLAB Function4/2(theta_dot_d)
  MATLAB Function3/1(theta_d) -> PID Controller (2DOF)2/1
  "q "/1 -> PID Controller (2DOF)3/2
  mass1/1 -> MATLAB Function3/3(mass)
  ang_st1/1 -> MATLAB Function4/1(angular_state)
  ang_st2/1 -> MATLAB Function6/1(angular_state)
  r/1 -> PID Controller (2DOF)5/2
  PID Controller/1 -> MATLAB Function6/2(psi_dot_d)
  MATLAB Function6/1(r_d) -> PID Controller (2DOF)5/1
  PID Controller (2DOF)3/1 -> Autopilot/2(q_dot_d)
  PID Controller (2DOF)5/1 -> Autopilot/3(r_dot_d)
  Aero_coffecients read1/1 -> Autopilot/6(aero_data)
  Structure_data_read/1 -> Autopilot/7(structure_data)
  Data Store Read2/1 -> Autopilot/8(Thrust)
  Clock/1 -> MATLAB Function1/1(t)
  Data Store Read1/1 -> MATLAB Function3/2(TT)
  Clock1/1 -> MATLAB Function3/1(t)
  Clock2/1 -> MATLAB Function5/1(t)
  u,v/1 -> Demux1/1
  Demux1/1 -> MATLAB Function5/2(u)
  Demux1/2 -> MATLAB Function5/3(v)
  MATLAB Function5/1(psi_d) -> MATLAB Function/1(psi_d)
  psi/1 -> MATLAB Function/2(psi)
  MATLAB Function/1(psi_error) -> PID Controller/1
  MATLAB Function7/1(u_dot_d) -> MATLAB Function3/4(a_x_d)
  MATLAB Function7/2(v_dot_d) -> MATLAB Function1/4(a_y_d)
  MATLAB Function7/3(w_dot_d) -> Terminator/1

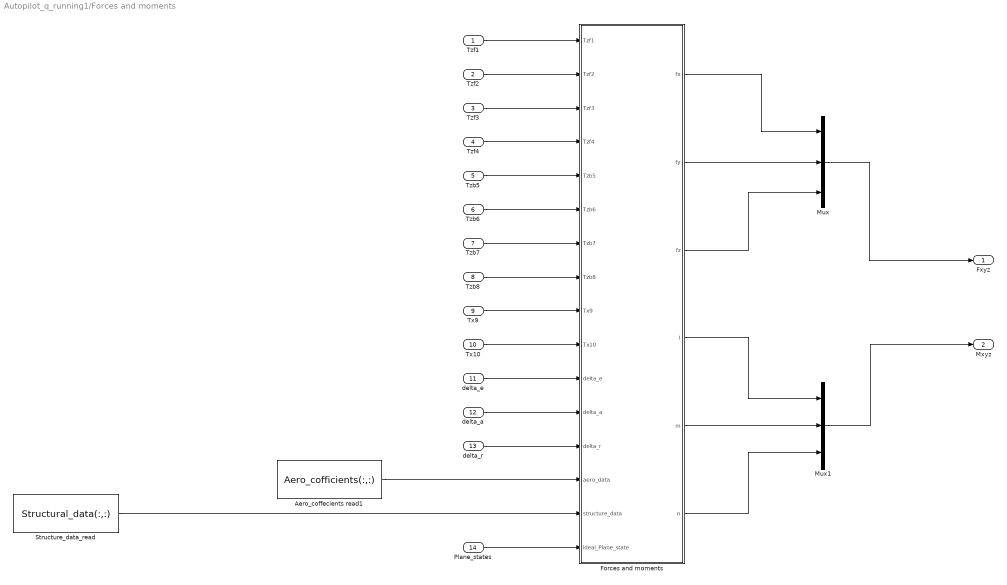
== system Autopilot_q_running1/Forces and moments ==
  Tzf1 : Inport
  Tzf2 : Inport  Port=2
  "Tzf3 " : Inport  Port=3
  Tzf4 : Inport  Port=4
  Tzb5 : Inport  Port=5
  Tzb6 : Inport  Port=6
  Tzb7 : Inport  Port=7
  Tzb8 : Inport  Port=8
  Tx9 : Inport  Port=9
  Tx10 : Inport  Port=10
  delta_e : Inport  Port=11
  delta_a : Inport  Port=12
  delta_r : Inport  Port=13
  Plane_states : Inport  Port=14
  Aero_coffecients read1 : DataStoreRead  DataStoreName=Aero_cofficients  DataStoreElements=Aero_cofficients(:,:)  IndexOptions=Index vector (dialog)  Indices=1  OutputSizes=1
  Forces and moments : MATLAB Function  TreatAsAtomicUnit=on
  Mux : Mux  Inputs=3
  Mux1 : Mux  Inputs=3
  Structure_data_read : DataStoreRead  DataStoreName=Structural_data  DataStoreElements=Structural_data(:,:)  IndexOptions=Index vector (dialog)  Indices=1  OutputSizes=1
  Fxyz : Outport  VectorParamsAs1DForOutWhenUnconnected=off
  Mxyz : Outport  Port=2  VectorParamsAs1DForOutWhenUnconnected=off
  wires:
  Tzf2/1 -> Forces and moments/2(Tzf2)
  Tzf1/1 -> Forces and moments/1(Tzf1)
  "Tzf3 "/1 -> Forces and moments/3(Tzf3)
  Tzf4/1 -> Forces and moments/4(Tzf4)
  Tzb5/1 -> Forces and moments/5(Tzb5)
  Tzb6/1 -> Forces and moments/6(Tzb6)
  Tzb7/1 -> Forces and moments/7(Tzb7)
  Tzb8/1 -> Forces and moments/8(Tzb8)
  Tx9/1 -> Forces and moments/9(Tx9)
  Tx10/1 -> Forces and moments/10(Tx10)
  delta_e/1 -> Forces and moments/11(delta_e)
  delta_a/1 -> Forces and moments/12(delta_a)
  delta_r/1 -> Forces and moments/13(delta_r)
  Forces and moments/1(fx) -> Mux/1
  Mux1/1 -> Mxyz/1
  Mux/1 -> Fxyz/1
  Forces and moments/2(fy) -> Mux/2
  Forces and moments/3(fz) -> Mux/3
  Forces and moments/4(l) -> Mux1/1
  Forces and moments/6(n) -> Mux1/3
  Forces and moments/5(m) -> Mux1/2
  Structure_data_read/1 -> Forces and moments/15(structure_data)
  Aero_coffecients read1/1 -> Forces and moments/14(aero_data)
  Plane_states/1 -> Forces and moments/16(ideal_Plane_state)
